simulink library "RGP_objF"  (R2018b)
settings: Solver=VariableStepAuto  StartTime=0.0  StopTime=10.0  RelTol=1e-3
libraries: simulink x2, dspsigops x1, RGP_objF_ul x1
settings Model: Creator=Ayaz  LastModifiedBy=Ayaz
settings DataIOCC: ReturnWorkspaceOutputs=on

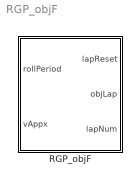
== system RGP_objF ==
  RGP_objF : Subsystem  mask{vRated=20}
      mask prompts: vRated "Turbine rated speed [cm/s]"
      mask TypeOptions vRated: Constant4/Value

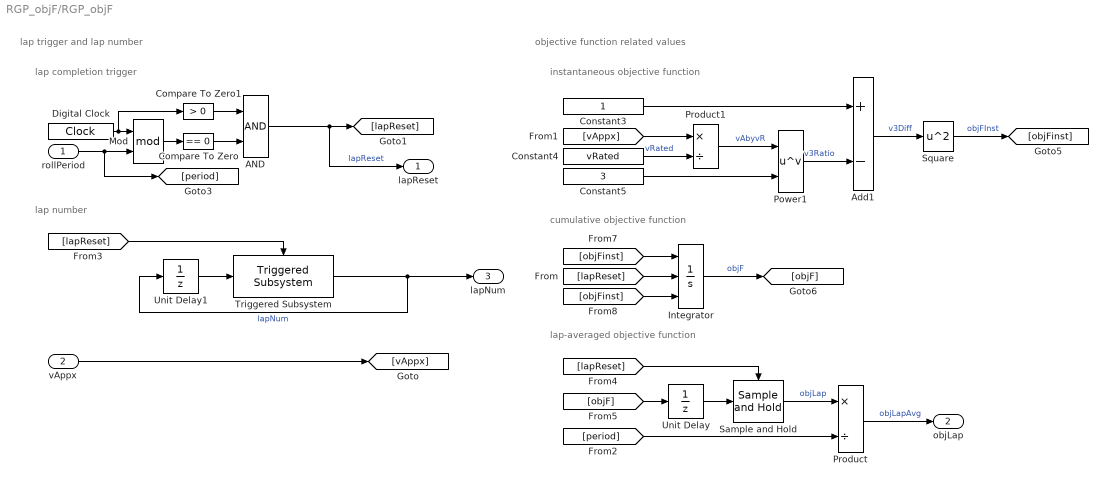
== system RGP_objF/RGP_objF ==
  note: instantaneous objective function
  note: lap completion trigger
  note: lap trigger and lap number
  note: objective function related values
  note: cumulative objective function
  note: lap number
  note: lap-averaged objective function
  rollPeriod : Inport
  vAppx : Inport  Port=2
  AND : Logic  AllPortsSameDT=off  OutDataTypeStr=boolean
  Add1 : Sum  Inputs=+-
  Compare To Zero : simulink/Logic and Bit Operations/Compare To Zero  relop===  OutDataTypeStr=boolean
  Compare To Zero1 : simulink/Logic and Bit Operations/Compare To Zero  relop=>  OutDataTypeStr=boolean
  Constant3 : Constant
  Constant4 : Constant  Value=vRated  VectorParams1D=off
  Constant5 : Constant  Value=3
  Digital Clock : DigitalClock
  Integrator : Integrator  ExternalReset=rising  InitialConditionSource=external
  Mod : Math  Operator=mod  SaturateOnIntegerOverflow=on
  Power1 : Math  Operator=pow  SaturateOnIntegerOverflow=on
  Product : Product  Inputs=*/
  Product1 : Product  Inputs=*/
  Sample and Hold : dspsigops/Sample and Hold  trig=Rising edge  initCond=0  latchinput=off
  Square : Math  Operator=square  SaturateOnIntegerOverflow=on
  Triggered Subsystem : RGP_objF_ul/RGP_objF/Triggered Subsystem  SystemSampleTime=-1  Latency=0  AutoFrameSizeCalculation=off
  Unit Delay : UnitDelay  SampleTime=-1  HasFrameUpgradeWarning=on
  Unit Delay1 : UnitDelay  SampleTime=-1  HasFrameUpgradeWarning=on
  lapReset : Outport
  objLap : Outport  Port=2
  lapNum : Outport  Port=3
  wires:
  [objFinst] -> Integrator/1
  Add1/1 -> Square/1  "v3Diff"
  Product1/1 -> Power1/1  "vAbyvR"
  Digital Clock/1 -> Compare To Zero1/1, Mod/1
  Square/1 -> [objFinst]  "objFInst"
  Power1/1 -> Add1/2  "v3Ratio"
  Unit Delay1/1 -> Triggered Subsystem/1
  [period] -> Product/2
  Mod/1 -> Compare To Zero/1
  Constant5/1 -> Power1/2
  rollPeriod/1 -> [period], Mod/2
  [objFinst] -> Integrator/3
  Integrator/1 -> [objF]  "objF"
  Product/1 -> objLap/1  "objLapAvg"
  AND/1 -> lapReset/1, [lapReset]  "lapReset"
  Constant3/1 -> Add1/1
  [lapReset] -> Triggered Subsystem/Trigger
  Sample and Hold/1 -> Product/1  "objLap"
  [objF] -> Unit Delay/1
  Unit Delay/1 -> Sample and Hold/1
  Compare To Zero/1 -> AND/2
  [lapReset] -> Sample and Hold/Trigger
  Triggered Subsystem/1 -> lapNum/1, Unit Delay1/1  "lapNum"
  [lapReset] -> Integrator/2
  Constant4/1 -> Product1/2  "vRated"
  [vAppx] -> Product1/1
  Compare To Zero1/1 -> AND/1
  vAppx/1 -> [vAppx]
